simulink model "ORC_test_simu_unregSCIG"  (R2018a)
settings: Solver=FixedStepAuto  StartTime=0.0  StopTime=10  FixedStep=.1  RelTol=1e-4
values from neighbouring files (symbols this model uses):
  A_cond = 50    [Chena_ORC_test_simu_init.m]    (also in ORC_test_simu_init.m = 18.6)
  A_evap = 30    [Chena_ORC_test_simu_init.m]    (also in ORC_test_simu_init.m = 9.3)
  Cx = 620e-05    (= 0.0062)    [Chena_ORC_test_simu_init.m]    (also in ORC_test_simu_init.m = 0.000221048532072; SCIG_Admittance_Balance.m = 6.9e-05; SCIG_Energy_Balance_excitation.m = 1.35135135135; SCIG_Energy_Balance_excitation_sym.m = 5)
  eff_inverter = 0.93    [Chena_ORC_test_simu_init.m]    (also in ORC_test_simu_init.m)
  eff_pump = 0.78    [Chena_ORC_test_simu_init.m]    (also in ORC_Energy_Balance.m = 0.7; ORC_test.m = 0.7; ORC_test_brownfield.m = 0.7; ORC_test_greenfield.m = 0.7)
  eff_turbine = 0.8    [Chena_ORC_test_simu_init.m]    (also in ORC_test_simu_init.m = 0.78)
  f_rated = 60    [Chena_ORC_test_simu_init.m]    (also in ORC_test_simu_init.m; SCIG_Admittance_Balance.m; SCIG_Admittance_test.m; SCIG_Ouazenne.m)
  H_wf_init = 2.6e+05    (= 260000)    [Chena_ORC_test_simu_init.m]    (also in ORC_test_simu_init.m = 230000)
  Lr = 0.252/(2*pi*f_rated)/35    (= 1.9098593171e-05)    [Chena_ORC_test_simu_init.m]    (also in ORC_test_simu_init.m = 0.000132629119243)
  Ls = 0.423/(2*pi*f_rated)/35    (= 3.20583528228e-05)    [Chena_ORC_test_simu_init.m]    (also in ORC_test_simu_init.m = 0.000848826363157)
  m_dot_source = 33.39    [Chena_ORC_test_simu_init.m]    (also in ORC_Energy_Balance.m = 5.7714; ORC_test.m = 12; ORC_test_brownfield.m = 6; ORC_test_greenfield.m = 12)
  m_dot_wf_init = 12    [Chena_ORC_test_simu_init.m]    (also in ORC_test_simu_init.m = 3)
  m_dot_wf_max = 16    [Chena_ORC_test_simu_init.m]
  magCurveV = [98.1532063054068,98.8036071709152,99.4518999785459,100.098037520928,100.741973127402,101.383660677656,102.023054614968,102.660109959042,103.294782318460,103.927027902737,104.556803533993,105.184066658235,105.808775356268,106.430888354220,107.050365033694,107.667165441552,108.281250299330,108.892581012284,109.501119678081,110.106829095126,110.709672770539,111.309614927775,111.906620513896,112.5006 ...(+6146 chars)    [Chena_ORC_test_simu_init.m]    (also in ORC_test_simu_init.m = [21.5410077151772,22.1687511430959,22.7961934111159,23.42344)
  magCurveX = [0.663529769645709,0.663521969965503,0.663500208426959,0.663464444749194,0.663414643227627,0.663350772676200,0.663272806369214,0.663180721982808,0.663074501536138,0.662954131332260,0.662819601898778,0.662670907928276,0.662508048218555,0.662331025612717,0.662139846939116,0.661934522951205,0.661715068267290,0.661481501310239,0.661233844247137,0.660972122928937,0.660696366830103,0.660406608988283,0.6 ...(+6531 chars)    [Chena_ORC_test_simu_init.m]    (also in ORC_test_simu_init.m = [21.5410077151772,21.5637559851946,21.5850104594817,21.60498)
  p_atm = 101325    [Chena_ORC_test_simu_init.m]    (also in ORC_test_simu_init.m)
  pf_grid = 0.9    [Chena_ORC_test_simu_init.m]    (also in ORC_test_simu_init.m)
  poles = 2    [Chena_ORC_test_simu_init.m]    (also in Copy_of_SCIG_Energy_Balance_excitation.m = 4; SCIG_Admittance_Balance.m = 6; SCIG_Admittance_test.m = 6; SCIG_Ouazenne.m)
  Rr = 0.144/35    (= 0.00411428571429)    [Chena_ORC_test_simu_init.m]    (also in ORC_test_simu_init.m = 0.03)
  Rs = 0.148/35    (= 0.00422857142857)    [Chena_ORC_test_simu_init.m]    (also in ORC_test_simu_init.m = 0.018)
  Rx = 0    [Chena_ORC_test_simu_init.m]    (also in Copy_of_SCIG_Energy_Balance_excitation.m = 0.003; ORC_test_simu_init.m; SCIG_Admittance_Balance.m; SCIG_Admittance_test.m)
  Tin_sink = 277.59    [Chena_ORC_test_simu_init.m]    (also in ORC_test_simu_init.m = 278)
  Tin_source = 346.48    [Chena_ORC_test_simu_init.m]    (also in ORC_test_simu_init.m = 368)
  U_cond = 5000    [Chena_ORC_test_simu_init.m]    (also in ORC_test_simu_init.m = 1400)
  U_evap = 4500    [Chena_ORC_test_simu_init.m]    (also in ORC_test_simu_init.m = 1500)
  Vline_rated = 220    [Chena_ORC_test_simu_init.m]    (also in SCIG_Admittance_Balance.m = 6600; SCIG_Admittance_test.m = 6600; SCIG_Ouazenne.m; SCIG_Ouazenne_iterate.m)
  Xx = 1/(2*pi*f_rated*Cx)    (= 0.427835868527)    [Chena_ORC_test_simu_init.m]    (also in Copy_of_SCIG_Energy_Balance_excitation.m = 12; ORC_test_simu_init.m = 12; SCIG_Admittance_Balance.m = Xx(fvIDX); SCIG_Energy_Balance_excitation.m = 1./(Cx.*w_synch))
undefined symbols (not defined in the file or in its folder): handle_sink, handle_source, handle_wf, n_mech_init, n_mech_max, n_mech_min, sigbuilder_block
(part 3 of 4)

== matlab function ORC_test_simu_unregSCIG/ORC/Condensor/HeatExNTU_3_cond ==
  data: T_or_H_hi input; P output; m_dot_h input; p_h input; T_or_H_ci input; m_dot_c input; p_c input; fluid_h parameter uint8; fluid_c parameter; HeatExType parameter; T_or_H_ho output; T_or_H_co output; U parameter; A parameter; T_or_H parameter boolean
function [ P, T_or_H_ho, T_or_H_co ] = HeatExNTU_3_block( T_or_H_hi, m_dot_h, p_h,  ...
    T_or_H_ci, m_dot_c, p_c, fluid_h, fluid_c, HeatExType, U, A, T_or_H )

%HeatExNTU Summary 
%   This function calculates flow and outlet temperatures of a heat exchanger
%   using the Number of Transfer Units (NTU) method as described in
%   Fundementals of Heat and Mass Transfer by F. P. Incropera, D. P.
%   DeWitt, T. L. Bergman & A. S. Lavine. The method can be used when only
%   the inlet tempertures are known as opposed to inlet and outlet
%   temperatures.
%
%   This is done by calculating effectiveness which is defined as the ratio
%   of actual heat transferred to the maximum possible heat transferred for 
%   an infinite length counter-flow heat exchanger with the given inlet
%   temperatures. The effectivenes is calculated differently depending on 
%   the geometry of exchanger but is always a function of the ratio of heat
%   capacity rates as well as the number of transfer units (NTU). The NTU
%   depends on the overall heat transfer coefficient, the heat transfer
%   area, and the smaller of the two heat capacity rates. 
%   
%   In the event of a phase change the rate of change of energy required to
%   get the fluid just beyond the point of vaporizaion or condensation is
%   calculated using the CoolProp function. Then the function is called
%   again at the new temperature and the final temperatures and heat rates
%   are calucluated using a reduced heat exhange area. I currently assume
%   the effected heat transfer area is a half of the original input. This 
%   function cannot accurately handle both fluids changing phase because it
%   does not check which fluid would change first.
% 
% Note: The effectiveness is separte from efficiency. The calculations
%   assumes an efficiency of 1 where all heat is transferred from the hot
%   fluid to the cool fluid or remains within the the fluid. This also
%   assumes no fluid is undergoing a change in state, which may not be
%   sufficient for my final model.
%
% This function makes use of CoolProp, a shared DLL. 
% More information about the Matlab wrapper can be found at
%   http://www.coolprop.org/coolprop/wrappers/MATLAB/index.html
% A list of parameters can be found at 
%   http://www.coolprop.org/coolprop/HighLevelAPI.html#parameter-table
% A list of fluids can be found at 
%   http://www.coolprop.org/fluid_properties/PurePseudoPure.html#list-of-fluids
%
% Inputs:
%   T_or_H_hi   Hot fluid inlet temperature in Kelvin or enthalpy in J/kg
%   m_dot_h     Hot fluid mass flow rate in kg/s
%   p_h         Hot fluid pressure in pa
%   fluid_h     Name of Hot fluid (string)
%   T_or_H_ci   Cool fluid inlet temperature in Kelvin or enthalpy in J/kg
%   m_dot_c     Cool fluid mass flow rate in kg/s
%   p_c         Cool fluid pressure in pa
%   fluid_c     Name of Cool fluid (string)
%   HeatExType  String describing the heat exchanger geometry. Currently
%               this variable only accepts 'counter' and 'parallel', but
%               can be expanded to other exchanger/flow types
%               'counter' for counter flow
%               'parallel' for parallel
%   U           Overall heat transfer coefficient in W/(K m2)
%   A           Heat transfer area in m2
%   T_or_H      String stating whether arguements 1&5 are temperature (T) 
%               or enthaply (H). Also applies to output
%
% Output:
%   P           Rate of heat exchenged (power) in W
%   T_or_H_ho   Hot fluid outlet temperature (K) or enthalpy J/kg
%   T_or_H_co   Cool fluid outlet temperature (K) or enthalpy J/kg

% initailize certain parameters used to call coolprop library
buffer_size = 255;
ierr = 0;
b = (1:1:buffer_size);
herr= char(b);
coder.extrinsic('calllib') 
coder.extrinsic('libpointer') 

% All the input signals should be the same size, so it shouldn't matter
% which one is used to obtain signal length
var_length = length(T_or_H_hi);
% T_or_H_hi

% fluid_h = 'water';
% fluid_c = 'R245fa';
% % initialize handles for hot and cool fluids
% [fluid_h, ~] = calllib('coolprop','AbstractState_factory',backend,fluid_h,ierr,herr,buffer_size);
% [fluid_c, ~] = calllib('coolprop','AbstractState_factory',backend,fluid_c,ierr,herr,buffer_size);

% determine input parameter pair indecies for coolprop calls
[pq_ind,~] = calllib('coolprop','get_input_pair_index','PQ_INPUTS'); %pressure and Mass vapor quality
[pt_ind,~] = calllib('coolprop','get_input_pair_index','PT_INPUTS'); %pressure and temperature
[hp_ind,~] = calllib('coolprop','get_input_pair_index','HmassP_INPUTS'); %Mass specific enthalpy and pressure

% determine output parameter indecies for coolprop calls
[t_ind, ~] = calllib('coolprop','get_param_index','T'); %temperature
[h_ind, ~] = calllib('coolprop','get_param_index','Hmass'); %Mass specific enthalpy
[c_ind, ~] = calllib('coolprop','get_param_index','Cpmass'); %Mass specific constant pressure specific heat

% find pointer location of pressure and temperature input values
p_h_Ptr = libpointer('doublePtr',p_h);
p_c_Ptr = libpointer('doublePtr',p_c);
% Thi_Ptr
% Tci_Ptr
% Hhi_Ptr
% Hci_Ptr

% initialize output to zeros of appropriate length. It is necessary to
% assign output variables before recursively calling this function.
T_or_H_ho = zeros(var_length,1);
T_or_H_co = zeros(var_length,1);
% P = zeros(size(T_or_H_hi));

% disp(T_or_H )
% Ensure temperature/enthalpy input variables are delt with appropriately
% if upper(T_or_H) == 'T' %|| 'TEMPERATURE'
if T_or_H %== 'T' %|| 'TEMPERATURE'
% Assume given temperature values are not at vaporization/condensation
% disp('Assuming Temperature input')
% Initialize T and H values 
    Thi = T_or_H_hi;
    Tci = T_or_H_ci;
    Thi_Ptr = libpointer('doublePtr',Thi);
    Tci_Ptr = libpointer('doublePtr',Tci);
    Hhi = zeros(var_length,1); % initialized to 0 temporarily
    Hci = zeros(var_length,1); % initialized to 0 temporarily
    Hhi_Ptr = libpointer('doublePtr',Hhi);
    Hci_Ptr = libpointer('doublePtr',Hci);
    
% Update values located at Hhi and Hci pointer locations
    calllib('coolprop','AbstractState_update_and_1_out', fluid_h, pt_ind, p_h_Ptr, Thi_Ptr, var_length, h_ind, Hhi_Ptr, ierr,herr,buffer_size);
    calllib('coolprop','AbstractState_update_and_1_out', fluid_c, pt_ind, p_c_Ptr, Tci_Ptr, var_length, h_ind, Hci_Ptr, ierr,herr,buffer_size);
% Set Hhi & Hci to values stored at pointer location
    Hhi = get(Hhi_Ptr,'Value');
    Hci = get(Hci_Ptr,'Value');

% elseif upper(T_or_H) == 'H' %|| 'ENTHALPY'
else%if T_or_H == 'H' %|| 'ENTHALPY'
% Enthalpy values can be in vaporization/condensation region    
% disp('Assuming Enthalpy input')
% Initialize H and T values
    Hhi = T_or_H_hi;
    Hci = T_or_H_ci;
    Hhi_Ptr = libpointer('doublePtr',Hhi);
    Hci_Ptr = libpointer('doublePtr',Hci);
    Thi = zeros(var_length,1); %initialized to 0 temporarily
    Tci = zeros(var_length,1); %initialized to 0 temporarily
    Thi_Ptr = libpointer('doublePtr',Thi);
    Tci_Ptr = libpointer('doublePtr',Tci);

% Update values located at Thi and Tci pointer locations
    calllib('coolprop','AbstractState_update_and_1_out', fluid_h, hp_ind, Hhi_Ptr, p_h_Ptr, var_length, t_ind, Thi_Ptr, ierr,herr,buffer_size);
    calllib('coolprop','AbstractState_update_and_1_out', fluid_c, hp_ind, Hci_Ptr, p_c_Ptr, var_length, t_ind, Tci_Ptr, ierr,herr,buffer_size);
% Set Thi & Tci to values stored at pointer location
    Thi = get(Thi_Ptr,'Value');
    Tci = get(Tci_Ptr,'Value');
    
% else
%     error('Please specify whether input uses variables of Temperature or Enthalpy.')
end
    

% Determine vaporization temperature for fluids at respective pressures.
% Initialize pointer locations for fluid quality and relevant temperatures
Q_Ptr = libpointer('doublePtr', zeros(var_length,1)); % Q is specifically set to 0
Tvh = zeros(var_length,1); % initialized to 0 temporarily
Tvc = zeros(var_length,1); % initialized to 0 temporarily
Tvh_Ptr = libpointer('doublePtr', Tvh);
Tvc_Ptr = libpointer('doublePtr', Tvc);

% Update values located at the Tvc & Tvh pointer locations for vaporization
% conditions
calllib('coolprop','AbstractState_update_and_1_out', fluid_h, pq_ind, p_h_Ptr, Q_Ptr, var_length, t_ind, Tvh_Ptr, ierr,herr,buffer_size);
calllib('coolprop','AbstractState_update_and_1_out', fluid_c, pq_ind, p_c_Ptr, Q_Ptr, var_length, t_ind, Tvc_Ptr, ierr,herr,buffer_size);

% Set Tvh & Tvc to values stored at pointer location
Tvh = get(Tvh_Ptr,'Value');
Tvc = get(Tvc_Ptr,'Value');

% Determine vaporization enthalpies for fluids at respective pressures
% Min enthalpies of vaporization region for hot and cool fluids (Q = 0)
Hvh_min = zeros(var_length,1); % initialized to 0 temporarily
Hvc_min = zeros(var_length,1); % initialized to 0 temporarily
Hvh_min_Ptr = libpointer('doublePtr',Hvh_min);
Hvc_min_Ptr = libpointer('doublePtr',Hvc_min);
    
% Update values located at Hvh_max and Hvc_max pointer locations
calllib('coolprop','AbstractState_update_and_1_out', fluid_h, pq_ind, p_h_Ptr, Q_Ptr, var_length, h_ind, Hvh_min_Ptr, ierr,herr,buffer_size);
calllib('coolprop','AbstractState_update_and_1_out', fluid_c, pq_ind, p_c_Ptr, Q_Ptr, var_length, h_ind, Hvc_min_Ptr, ierr,herr,buffer_size);
% Set Hvh_max & Hvc_max to values stored at pointer location
Hvh_min = get(Hvh_min_Ptr,'Value');
Hvc_min = get(Hvc_min_Ptr,'Value');

% Max enthalpies of vaporization region for hot and cool fluid (Q = 1)
Q_Ptr = libpointer('doublePtr', ones(var_length,1)); % Q is specifically set to 1
Hvh_max = zeros(var_length,1); % initialized to 0 temporarily
Hvc_max = zeros(var_length,1); % initialized to 0 temporarily
Hvh_max_Ptr = libpointer('doublePtr',Hvh_max);
Hvc_max_Ptr = libpointer('doublePtr',Hvc_max);
    
% Update values located at Hvh_max and Hvc_max pointer locations
calllib('coolprop','AbstractState_update_and_1_out', fluid_h, pq_ind, p_h_Ptr, Q_Ptr, var_length, h_ind, Hvh_max_Ptr, ierr,herr,buffer_size);
calllib('coolprop','AbstractState_update_and_1_out', fluid_c, pq_ind, p_c_Ptr, Q_Ptr, var_length, h_ind, Hvc_max_Ptr, ierr,herr,buffer_size);
% Set Hvh_max & Hvc_max to values stored at pointer location
Hvh_max = get(Hvh_max_Ptr,'Value');
Hvc_max = get(Hvc_max_Ptr,'Value');


% Determine the specific heats of the incoming fluids using coolprop
% Initialize pointer locations for relevant variables
Ch = zeros(var_length,1); % initialized to 0 temporarily
Cc = zeros(var_length,1); % initialized to 0 temporarily
Ch_Ptr = libpointer('doublePtr', Ch); 
Cc_Ptr = libpointer('doublePtr', Cc); 

% Update values located at the Ch & Cc pointer locations for input
% conditions
calllib('coolprop','AbstractState_update_and_1_out', fluid_h, hp_ind, Hhi_Ptr, p_h_Ptr, var_length, c_ind, Ch_Ptr, ierr,herr,buffer_size);
calllib('coolprop','AbstractState_update_and_1_out', fluid_c, hp_ind, Hci_Ptr, p_c_Ptr, var_length, c_ind, Cc_Ptr, ierr,herr,buffer_size);

% Set Ch & Cc to values stored at pointer location
Ch = get(Ch_Ptr,'Value');   % J/(kg K)
Cc = get(Cc_Ptr,'Value');   % J/(kg K)

% If the fluid is withing the vaporization range then the coolprop library 
% will return an inaccurate values. If that happens then the specific heat 
% will be set to inf so its temperature will not change even though heat is
% exchanged.
Ch(Hhi <= Hvh_max & Hhi > Hvh_min) = inf;    % J/(kg K)
Cc(Hci < Hvc_max & Hci >= Hvc_min) = inf;    % J/(kg K)

% Calculate the heat capacity rates of the hot and cool fluids
Ch_rate = Ch .* m_dot_h;     % W/K
Cc_rate = Cc .* m_dot_c;     % W/K

% Determine the maximum and minimum of the two heat capacity rates
Cmax = Ch_rate; % W/K
Cmax(Ch_rate < Cc_rate) = Cc_rate(Ch_rate < Cc_rate);   % W/K
Cmin = Ch_rate; % W/K
Cmin(Ch_rate > Cc_rate) = Cc_rate(Ch_rate > Cc_rate);   % W/K

% Calcluate the heat capacity rate ratio 
Cr = Cmin./Cmax;

% unitA is the size of heat exchanger area(m2) each iteration of the script
% uses for calculating NTU
% unitA = 1;
unitA = A .* ones(var_length,1);

% Calculate the number of transfer units of the heat exchanger
if any(A < unitA)
    unitA = A .* ones(var_length,1);
%     NTU = U * A / Cmin
end

NTU = U * unitA ./ Cmin;


HeatExType = 'counter';
% Calculate effectiveness based on type of heat exchanger
switch HeatExType
    case 'counter'  % If the heat exchanger is counter-flow
        effectiveness = (1 - exp(-NTU.*(1 - Cr))) ./ ...
                        (1 - Cr.*exp(-NTU.*(1 - Cr)));
    case 'parallel' % If the heat exchanger is parallel-flow
        effectiveness = (1 - exp(-NTU.*(1 + Cr))) ./ ...
                        (1 + Cr);
    otherwise       % If not exchanger specified
%         warning('No heat exchanger type specified, therefore no heat is exchanged.')
        effectiveness = 0;
end        

% % However if the Cr is 0 (Cmax is inf) then effectiveness is calcluated
% % regardless of the heat exchanger flow.
% if Cr == 0
%     effectiveness = 1 - exp(-NTU);
% end
% effectiveness;


% Maximum energy transfer rate is equal for an infinite length heat
% exchanger is equal to Cmin multiplied with the difference in inlet
% temperatures. The actual energy transfer rate is the maximum rate
% multiplied by the effectiveness (Assuming no heat loss).
P = effectiveness.*Cmin.*(Thi - Tci);

% The change in temperature is calculated for both sides by dividing the
% energy tranfer rate by the heat capacity rates for both sides. This
% assumes the energy transfer rate is the same for both sides.
deltaTh = P./Ch_rate;
deltaTc = P./Cc_rate;

% The outlet temperatures are caluctaed by subtracting the change in
% temperature from the hot fluid inlet temperature and adding the change in
% temperature from the cool fluid inlet temperature.
Tho = Thi - deltaTh;
Tco = Tci + deltaTc;

% Determine Hho and Hco values based off of Tho and Tco values
% Initialize Hho and Hco values and pointers and Tho & Tco pointers
Tho_Ptr = libpointer('doublePtr',Tho);
Tco_Ptr = libpointer('doublePtr',Tco);
Hho = zeros(var_length,1); % initialized to 0 temporarily
Hco = zeros(var_length,1); % initialized to 0 temporarily
Hho_Ptr = libpointer('doublePtr',Hho);
Hco_Ptr = libpointer('doublePtr',Hco);
    
% Update values located at Hho and Hco pointer locations
calllib('coolprop','AbstractState_update_and_1_out', fluid_h, pt_ind, p_h_Ptr, Tho_Ptr, var_length, h_ind, Hho_Ptr, ierr,herr,buffer_size);
calllib('coolprop','AbstractState_update_and_1_out', fluid_c, pt_ind, p_c_Ptr, Tco_Ptr, var_length, h_ind, Hco_Ptr, ierr,herr,buffer_size);
% Set Hho & Hco to values stored at pointer location
Hho = get(Hho_Ptr,'Value');
Hco = get(Hco_Ptr,'Value');

% The coolprop will fail to update if Tho = vaporization temperature. In
% that case, those values will remain zero because it was initialized to 
% zero. For those values Ho = Hi - P/m_dot
Hho(~Hho) =  Hhi(~Hho) - P(~Hho)./m_dot_h(~Hho);

% The coolprop will fail to update if Tco = vaporization temperature. In
% that case, those values will remain zero because it was initialized to 
% zero. For those values Ho = Hi + P/m_dot
Hco(~Hco) =  Hci(~Hco) + P(~Hco)./m_dot_c(~Hco);


% check if hot fluid begins to condense 
if any(Hho <= Hvh_max & Hhi > Hvh_max)
% if Tho <= Tvh && Thi >= Tvh
%     disp('~~~~~~~~~~~~~~~~~~~Condensation start~~~~~~~~~~~~~~~~~~~~~')

%     Get the indecies where condensation starts
    cond_start_ind = (Hho <= Hvh_max & Hhi > Hvh_max);
    
%     Set the H output of the appropriate values to maximum value in the
%     vaporization region (Q = 1)
    Hho(cond_start_ind) = Hvh_max(cond_start_ind);
    Tho(cond_start_ind) = Tvh(cond_start_ind);
    
%     Calculate power needed to bring hot fluid initial state to
%     precondense for only relevant values
    P_init_to_precondense = (Hhi(cond_start_ind) - Hho(cond_start_ind)).*m_dot_h(cond_start_ind);

%     Calculate change in temperature for relavent cool fluid values
    deltaTc = P_init_to_precondense./Cc_rate(cond_start_ind);
%     Update relavent cool fluid output temperatures and get new pointer
    Tco(cond_start_ind) = Tci(cond_start_ind) + deltaTc;
    Tco_Ptr = libpointer('doublePtr',Tco);
    
%     Update H values for new cool output temperatures
    calllib('coolprop','AbstractState_update_and_1_out', fluid_c, pt_ind, p_c_Ptr, Tco_Ptr, var_length, h_ind, Hco_Ptr, ierr,herr,buffer_size);
    Hco = get(Hco_Ptr,'Value');

%     Calculate ratio of power to precondense state relative to initally
%     calculated power in order to correct the area of relavent values
    PowerFrac_Condense_over_NoCondense = P_init_to_precondense./P(cond_start_ind);
    unitA(cond_start_ind) = unitA(cond_start_ind)*PowerFrac_Condense_over_NoCondense;
%     Update relevant power values
    P(cond_start_ind) = P_init_to_precondense;
    
% check if hot fluid finishes condensing    
elseif any(Hho <= Hvh_min & Hhi > Hvh_min)
% elseif Tho <= Tvh && Thi >= Tvh
%     disp('~~~~~~~~~~~~~~~~~~~~~~Condensation end~~~~~~~~~~~~~~~~~~~~~~~~~')

%     Get the indecies where condensation starts
    cond_end_ind = (Hho <= Hvh_min & Hhi > Hvh_min);
    
%     Set the H output of the appropriate values to minimum value in the
%     vaporization region (Q = 0)
    Hho(cond_end_ind) = Hvh_min(cond_end_ind);
    Tho(cond_end_ind) = Tvh(cond_end_ind) - 1e-4;
    
%     Calculate power needed to bring hot fluid initial state to
%     postcondense for only relevant values
    P_init_to_postcondense = (Hhi(cond_end_ind) - Hho(cond_end_ind)).*m_dot_h(cond_end_ind);

%     Calculate change in temperature for relavent cool fluid values
    deltaTc = P_init_to_postcondense./Cc_rate(cond_end_ind);
%     Update relavent cool fluid output temperatures and get new pointer
    Tco(cond_end_ind) = Tci(cond_end_ind) + deltaTc;
    Tco_Ptr = libpointer('doublePtr',Tco);

%     Update H values for new cool output temperatures
    calllib('coolprop','AbstractState_update_and_1_out', fluid_c, pt_ind, p_c_Ptr, Tco_Ptr, var_length, h_ind, Hco_Ptr, ierr,herr,buffer_size);
    Hco = get(Hco_Ptr,'Value');

%     Calculate ratio of power to postcondense state relative to initally
%     calculated power in order to correct the area of relavent values
    PowerFrac_Condense_over_NoCondense = P_init_to_postcondense./P(cond_end_ind);
    unitA(cond_end_ind) = unitA(cond_end_ind)*PowerFrac_Condense_over_NoCondense;
%     Update relevant power values
    P(cond_end_ind) = P_init_to_postcondense;
 

% else check if cool fluid begins to vaporize
elseif any(Hco >= Hvc_min & Hci < Hvc_min)
% elseif Tco >= Tvc && Tci <= Tvc
%    disp('~~~~~~~~~~~~~~~~~~~Vaporization start~~~~~~~~~~~~~~~~~~~~~~~~')

%     Get the indecies where vaporization starts
    vap_start_ind = (Hco >= Hvc_min & Hci < Hvc_min);

%     Set the H output of the appropriate values to minimum value in the
%     vaporization region (Q = 0)
    Hco(vap_start_ind) = Hvc_min(vap_start_ind);
    Tco(vap_start_ind) = Tvc(vap_start_ind);

%     Calculate power needed to bring cool fluid initial state to
%     prevaporization for only relevant values
    P_init_to_prevap = (Hco(vap_start_ind) - Hci(vap_start_ind)).*m_dot_c(vap_start_ind);

%     Calculate change in temperature for relavent hot fluid values
    deltaTh = P_init_to_prevap./Ch_rate(vap_start_ind);
%     Update relavent hot fluid output temperatures and get new pointer
    Tho(vap_start_ind) = Thi(vap_start_ind) - deltaTh;
    Tho_Ptr = libpointer('doublePtr',Tho);

%     Update H values for new hot output temperatures
    calllib('coolprop','AbstractState_update_and_1_out', fluid_h, pt_ind, p_h_Ptr, Tho_Ptr, var_length, h_ind, Hho_Ptr, ierr,herr,buffer_size);
    Hho = get(Hho_Ptr,'Value');

%     Calculate ratio of power to prevaporize state relative to initally
%     calculated power in order to correct the area of relavent values
    PowerFrac_Vaporize_over_NoVaporize = P_init_to_prevap./P(vap_start_ind);
    unitA(vap_start_ind) = unitA(vap_start_ind).*PowerFrac_Vaporize_over_NoVaporize;
%     Update relevant power values
    P(vap_start_ind) = P_init_to_prevap;

    
% check if cool fluid finishes vaporizing
elseif any(Hco >= Hvc_max & Hci < Hvc_max)
% elseif Tho <= Tvh && Thi >= Tvh
%     disp('~~~~~~~~~~~~~~~~Vaporization end~~~~~~~~~~~~~~~~~~~~')

%     Get the indecies where vaporization ends
    vap_end_ind = (Hco >= Hvc_max & Hci < Hvc_max);

%     Set the H output of the appropriate values to maximum value in the
%     vaporization region (Q = 1)
    Hco(vap_end_ind) = Hvc_max(vap_end_ind);
    Tco(vap_end_ind) = Tvc(vap_end_ind) + 1e-4;

%     Calculate power needed to bring cool fluid initial state to
%     postvaporization for only relevant values
    P_init_to_postvap = (Hco(vap_end_ind) - Hci(vap_end_ind)).*m_dot_c(vap_end_ind);

%     Calculate change in temperature for relavent hot fluid values
    deltaTh = P_init_to_postvap./Ch_rate(vap_end_ind);
%     Update relavent hot fluid output temperatures and get new pointer
    Tho(vap_end_ind) = Thi(vap_end_ind) - deltaTh;
    Tho_Ptr = libpointer('doublePtr',Tho);

%     Update H values for new hot output temperatures
    calllib('coolprop','AbstractState_update_and_1_out', fluid_h, pt_ind, p_h_Ptr, Tho_Ptr, var_length, h_ind, Hho_Ptr, ierr,herr,buffer_size);
    Hho = get(Hho_Ptr,'Value');

%     Calculate ratio of power to prevaporize state relative to initally
%     calculated power in order to correct the area of relavent values
    PowerFrac_Vaporize_over_NoVaporize = P_init_to_postvap./P(vap_end_ind);
    unitA(vap_end_ind) = unitA(vap_end_ind).*PowerFrac_Vaporize_over_NoVaporize;
%     Update relevant power values
    P(vap_end_ind) = P_init_to_postvap;

else
%     disp('~~~~~~~~~~~~~~~~Maintain State~~~~~~~~~~~~~~~~~~~~')
end
%     Hhi
%     Hho
%     Thi
%     Tho
%     Hci
%     Hco
%     Tci
%     Tco
%     P

% double check if hot fluid would condense and cool fluid would vaporize
if any((Tho < Tvh & Thi > Tvh) & (Tco > Tvc & Tci < Tvc))
    error('This function cannot accurately handle both fluids changing phase.')
end

if A > unitA

%     P_next = zeros(size(T_or_H_hi));
%     disp(P)
    [ P_next, Hho, Hco ] = HeatExNTU_3_low( Hho, m_dot_h, p_h, ...
        Hco, m_dot_c, p_c, fluid_h, fluid_c, HeatExType, U, A - unitA, 'H' );
%     A
%     unitA
% %     A - unitA;
%     P_next
    P = P + P_next;
%     disp(['Power After: ' num2str(P) ' W'])

    Hho_Ptr = libpointer('doublePtr',Hho);
    Hco_Ptr = libpointer('doublePtr',Hco);
% Update values located at Tho and Tco pointer locations
    calllib('coolprop','AbstractState_update_and_1_out', fluid_h, hp_ind, Hho_Ptr, p_h_Ptr, var_length, t_ind, Tho_Ptr, ierr,herr,buffer_size);
    calllib('coolprop','AbstractState_update_and_1_out', fluid_c, hp_ind, Hco_Ptr, p_c_Ptr, var_length, t_ind, Tco_Ptr, ierr,herr,buffer_size);
% Set Thi & Tci to values stored at pointer location
    Tho = get(Tho_Ptr,'Value');
    Tco = get(Tco_Ptr,'Value');

else
%     P
end


% % Free the hot and cool fluid handles
% calllib('coolprop','AbstractState_free', fluid_h, ierr,herr,buffer_size);
% calllib('coolprop','AbstractState_free', fluid_c, ierr,herr,buffer_size);

% if upper(T_or_H) == 'T' %|| 'TEMPERATURE'
if T_or_H% == 'T' %|| 'TEMPERATURE'
    T_or_H_ho = Tho;
    T_or_H_co = Tco;
% elseif upper(T_or_H) == 'H' %|| 'ENTHALPY'
else%if T_or_H == 'H' %|| 'ENTHALPY'
    T_or_H_ho = Hho;
    T_or_H_co = Hco;
end
end

== matlab function ORC_test_simu_unregSCIG/ORC/Pump/IsentropicPower_pump ==
  data: T_or_H_i input; P_hy output; p_i input; p_o input; m_dot input; T_or_H_o output; T_or_H parameter; isen_eff parameter; fluid parameter
function [ P_hy, T_or_H_o ] = IsentropicPower_block( T_or_H_i, p_i, p_o, m_dot, T_or_H,  isen_eff, fluid)
% function [ P_hy ] = IsentropicPower( T_i, T_o, p_i, p_o, m_dot, fluid, isen_eff )
%EXPANDER Summary of this function
%   This process calculates the mechanical power provided or required by a 
%   generic expander device/system. Turbines and other expanders provide
%   mechanical power while pumps and compressors consume it. This is done
%   by calculating the change in enthalpy of fluid and multipying by the 
%   mass flow rate while entropy remains constant.  Non ideal processes are
%   taken into account through the isentropic efficiency.
% 
% Inputs:
%   T_or_H_i    Input temperature in Kelvin or enthalpy in J/kg
%   p_i         Input pressure of the fluid in Pa
%   p_o         Output temperature of the fluid in Pa
%   m_dot       Mass flow rate of the fluid in kg/s 
%   fluid       Initialzed coolprop fluid handle
%   isen_eff    Isentropic efficiency of the device. Expected range: 0-1
%               This input is optional. If it is not provided then it will 
%               be set to 1, which is the efficiency of an ideal isentropic
%               device where entropy is constant.
%               This value is treated differently depending on if there is
%               an increase or decrease in fluid enthalpy. If the enthalpy
%               decreases (energy is extracted from the system) then the
%               efficiency if multiplied by the change in energy because
%               less energy is extracted than the ideal case. If the
%               enthalpy increases (energy in added to the system) then the
%               efficiency is divided by the change in energy because more
%               energy is required than the ideal case.
%   T_or_H      Logical indicating whether the relavent input and output
%               variables are temperature (1) or enthalpy (0)
% 
% Outputs:
%   P_hy        Hydraulic power exctracted or consumed in W. Positive
%               values indicate the system is providing hydraulic power as
%               a turbine or expander. Negative values indicate the system 
%               is consuming hydraulic power as a compressor or pump.
%   T_or_H_o    Output temperature in Kelvin or enthalpy in J/kg

% This function makes use of the CoolProp wrapper for fluid properties. 
% The high level Matlab wrapper cannot handle vector inputs. There ways to
% make low level calls interfacing with the DLL so many values can be
% determined more quickly, but that is not implented here.
% More information about the Matlab wrapper can be found at
%   http://www.coolprop.org/coolprop/wrappers/MATLAB/index.html
% A list of parameters can be found at 
%   http://www.coolprop.org/coolprop/HighLevelAPI.html#parameter-table
% A list of fluids can be found at 
%   http://www.coolprop.org/fluid_properties/PurePseudoPure.html#list-of-fluids

% initailize certain parameters used to call coolprop library
buffer_size = 255;
ierr = 0;
b = (1:1:buffer_size);
herr= char(b);
coder.extrinsic('calllib') 
coder.extrinsic('libpointer') 

% All the input signals should be the same size, so it shouldn't matter
% which one is used to obtain signal length
var_length = length(T_or_H_i);

% determine input parameter pair indecies for coolprop calls
% [pq_ind,~] = calllib('coolprop','get_input_pair_index','PQ_INPUTS'); %pressure and Mass vapor quality
[pt_ind,~] = calllib('coolprop','get_input_pair_index','PT_INPUTS'); %pressure and temperature
[hp_ind,~] = calllib('coolprop','get_input_pair_index','HmassP_INPUTS'); %Mass specific enthalpy and pressure
[ps_ind,~] = calllib('coolprop','get_input_pair_index','PSmass_INPUTS'); %pressure and Mass specific entropy

% determine output parameter indecies for coolprop calls
[t_ind, ~] = calllib('coolprop','get_param_index','T'); %temperature
[s_ind, ~] = calllib('coolprop','get_param_index','S'); %Mass specific entropy
[h_ind, ~] = calllib('coolprop','get_param_index','Hmass'); %Mass specific enthalpy
% [c_ind, ~] = calllib('coolprop','get_param_index','Cpmass'); %Mass specific constant pressure specific heat

% find pointer location of pressure input and output values
p_i_Ptr = libpointer('doublePtr',p_i);
p_o_Ptr = libpointer('doublePtr',p_o);

% Ensure temperature/enthalpy input variables are delt with appropriately
if T_or_H 
% Assume given temperature values are not at vaporization/condensation.
% Initialize T and H inputs
    T_i = T_or_H_i;
    T_i_Ptr = libpointer('doublePtr',T_i);
    H_i = zeros(var_length,1); % initialized to 0 temporarily
    H_i_Ptr = libpointer('doublePtr',H_i);
% Update values located at Hhi and Hci pointer locations
    calllib('coolprop','AbstractState_update_and_1_out', fluid, pt_ind, p_i_Ptr, T_i_Ptr, var_length, h_ind, H_i_Ptr, ierr,herr,buffer_size);
% Set Hhi & Hci to values stored at pointer location
    H_i = get(H_i_Ptr,'Value');
    
else
% Enthalpy values can be in vaporization/condensation region  
% Initialize H values
    H_i = T_or_H_i;
    H_i_Ptr = libpointer('doublePtr',H_i);

end

% Input entropy in J/kg/K
% Initialize pointer locations for relevant variables
S_i_Ptr = libpointer('doublePtr', zeros(var_length,1)); 
% Update values at S_i pointer location
calllib('coolprop','AbstractState_update_and_1_out', fluid, hp_ind, H_i_Ptr, p_i_Ptr, var_length, s_ind, S_i_Ptr, ierr,herr,buffer_size);
% Set S_i to values stored at pointer location
% S_i = get(S_i_Ptr,'Value');

% Ideal Output entropy is equal to input entropy 
% Ideal Output enthalpy in J/kg and temperature
H_o_ideal = zeros(var_length,1);
H_o_ideal_Ptr = libpointer('doublePtr',H_o_ideal);
% Update values located at Hhi and Hci pointer locations
calllib('coolprop','AbstractState_update_and_1_out', fluid, ps_ind, p_o_Ptr, S_i_Ptr, var_length, h_ind, H_o_ideal_Ptr, ierr,herr,buffer_size);
% Set H_o_ideal to values stored at pointer location
H_o_ideal = get(H_o_ideal_Ptr,'Value');

% Calculate Ideal power consumed/provided
P_ideal = m_dot.*(H_i - H_o_ideal);

% Initialize hydrolic power variable
P_hy = zeros(var_length,1);
%   If positive then the system is providing power as a turbine
%   or expander.
%   This means the actual power provided is less than the ideal power
P_hy(P_ideal > 0) = isen_eff.*P_ideal(P_ideal > 0);

%   If negative then the system is consuming power as a
%   compressor or pump.
%   This means the actual power consumed is greater than the ideal power.
P_hy(P_ideal < 0) = P_ideal(P_ideal < 0)./isen_eff;

% Set output enthalpy
H_o = H_i - P_hy./m_dot;
H_o_Ptr = libpointer('doublePtr',H_o);

% Ensure temperature/enthalpy input variables are delt with appropriately
if T_or_H 
% Assume given temperature values are not at vaporization/condensation
    T_or_H_o = zeros(var_length,1);
    T_or_H_o_Ptr = libpointer('doublePtr',T_or_H_o);
    calllib('coolprop','AbstractState_update_and_1_out', fluid, hp_ind, H_o_Ptr, p_o_Ptr, var_length, t_ind, T_or_H_o_Ptr, ierr,herr,buffer_size);
    T_or_H_o = get(T_or_H_o_Ptr,'Value');
    
else
% Enthalpy values can be in vaporization/condensation region    
    T_or_H_o = H_o;
end
end

== matlab function ORC_test_simu_unregSCIG/ORC/hp2t ==
  data: temperature output; enthalpy input; pressure input; fluid_handle parameter
function temperature  = hp2t(enthalpy,pressure, fluid_handle)
%HP2T Summary of this function goes here
%   This function takes caluculates the temperature of a fluid based off of
%   its enthalpy and pressure using the Cool Prob library. The fluid handle
%   must already be generated and input in order to calculate the output
%   values.

buffer_size = 255;
ierr = 0;
b = (1:1:buffer_size);
herr= char(b);
coder.extrinsic('calllib') 
coder.extrinsic('libpointer') 

[hp_ind,~] = calllib('coolprop','get_input_pair_index','HmassP_INPUTS'); %Mass specific enthalpy and pressure
[t_ind, ~] = calllib('coolprop','get_param_index','T'); %temperature

var_len = length(pressure);
pressurePtr = libpointer('doublePtr',pressure);
enthaplyPtr = libpointer('doublePtr',enthalpy);
temperature = zeros(var_len,1);
temperaturePtr = libpointer('doublePtr',temperature);

calllib('coolprop','AbstractState_update_and_1_out', fluid_handle, hp_ind, enthaplyPtr, pressurePtr, var_len, t_ind, temperaturePtr, ierr,herr,buffer_size);

temperature = get(temperaturePtr,'Value');

end

== matlab function ORC_test_simu_unregSCIG/ORC/hp2t1 ==
  data: temperature output; enthalpy input; pressure input; fluid_handle parameter
function temperature  = hp2t(enthalpy,pressure, fluid_handle)
%HP2T Summary of this function goes here
%   This function takes caluculates the temperature of a fluid based off of
%   its enthalpy and pressure using the Cool Prob library. The fluid handle
%   must already be generated and input in order to calculate the output
%   values.

buffer_size = 255;
ierr = 0;
b = (1:1:buffer_size);
herr= char(b);
coder.extrinsic('calllib') 
coder.extrinsic('libpointer') 

[hp_ind,~] = calllib('coolprop','get_input_pair_index','HmassP_INPUTS'); %Mass specific enthalpy and pressure
[t_ind, ~] = calllib('coolprop','get_param_index','T'); %temperature

var_len = length(pressure);
pressurePtr = libpointer('doublePtr',pressure);
enthaplyPtr = libpointer('doublePtr',enthalpy);
temperature = zeros(var_len,1);
temperaturePtr = libpointer('doublePtr',temperature);

calllib('coolprop','AbstractState_update_and_1_out', fluid_handle, hp_ind, enthaplyPtr, pressurePtr, var_len, t_ind, temperaturePtr, ierr,herr,buffer_size);

temperature = get(temperaturePtr,'Value');

end

== matlab function ORC_test_simu_unregSCIG/ORC/hp2t2 ==
  data: temperature output; enthalpy input; pressure input; fluid_handle parameter
function temperature  = hp2t(enthalpy,pressure, fluid_handle)
%HP2T Summary of this function goes here
%   This function takes caluculates the temperature of a fluid based off of
%   its enthalpy and pressure using the Cool Prob library. The fluid handle
%   must already be generated and input in order to calculate the output
%   values.

buffer_size = 255;
ierr = 0;
b = (1:1:buffer_size);
herr= char(b);
coder.extrinsic('calllib') 
coder.extrinsic('libpointer') 

[hp_ind,~] = calllib('coolprop','get_input_pair_index','HmassP_INPUTS'); %Mass specific enthalpy and pressure
[t_ind, ~] = calllib('coolprop','get_param_index','T'); %temperature

var_len = length(pressure);
pressurePtr = libpointer('doublePtr',pressure);
enthaplyPtr = libpointer('doublePtr',enthalpy);
temperature = zeros(var_len,1);
temperaturePtr = libpointer('doublePtr',temperature);

calllib('coolprop','AbstractState_update_and_1_out', fluid_handle, hp_ind, enthaplyPtr, pressurePtr, var_len, t_ind, temperaturePtr, ierr,herr,buffer_size);

temperature = get(temperaturePtr,'Value');

end

== matlab function ORC_test_simu_unregSCIG/ORC/hp2t3 ==
  data: temperature output; enthalpy input; pressure input; fluid_handle parameter
function temperature  = hp2t(enthalpy,pressure, fluid_handle)
%HP2T Summary of this function goes here
%   This function takes caluculates the temperature of a fluid based off of
%   its enthalpy and pressure using the Cool Prob library. The fluid handle
%   must already be generated and input in order to calculate the output
%   values.

buffer_size = 255;
ierr = 0;
b = (1:1:buffer_size);
herr= char(b);
coder.extrinsic('calllib') 
coder.extrinsic('libpointer') 

[hp_ind,~] = calllib('coolprop','get_input_pair_index','HmassP_INPUTS'); %Mass specific enthalpy and pressure
[t_ind, ~] = calllib('coolprop','get_param_index','T'); %temperature

var_len = length(pressure);
pressurePtr = libpointer('doublePtr',pressure);
enthaplyPtr = libpointer('doublePtr',enthalpy);
temperature = zeros(var_len,1);
temperaturePtr = libpointer('doublePtr',temperature);

calllib('coolprop','AbstractState_update_and_1_out', fluid_handle, hp_ind, enthaplyPtr, pressurePtr, var_len, t_ind, temperaturePtr, ierr,herr,buffer_size);

temperature = get(temperaturePtr,'Value');

end

== matlab function ORC_test_simu_unregSCIG/ORC/hp2t4 ==
  data: temperature output; enthalpy input; pressure input; fluid_handle parameter
function temperature  = hp2t(enthalpy,pressure, fluid_handle)
%HP2T Summary of this function goes here
%   This function takes caluculates the temperature of a fluid based off of
%   its enthalpy and pressure using the Cool Prob library. The fluid handle
%   must already be generated and input in order to calculate the output
%   values.

buffer_size = 255;
ierr = 0;
b = (1:1:buffer_size);
herr= char(b);
coder.extrinsic('calllib') 
coder.extrinsic('libpointer') 

[hp_ind,~] = calllib('coolprop','get_input_pair_index','HmassP_INPUTS'); %Mass specific enthalpy and pressure
[t_ind, ~] = calllib('coolprop','get_param_index','T'); %temperature

var_len = length(pressure);
pressurePtr = libpointer('doublePtr',pressure);
enthaplyPtr = libpointer('doublePtr',enthalpy);
temperature = zeros(var_len,1);
temperaturePtr = libpointer('doublePtr',temperature);

calllib('coolprop','AbstractState_update_and_1_out', fluid_handle, hp_ind, enthaplyPtr, pressurePtr, var_len, t_ind, temperaturePtr, ierr,herr,buffer_size);

temperature = get(temperaturePtr,'Value');

end

== matlab function ORC_test_simu_unregSCIG/ORC/hp2t5 ==
  data: temperature output; enthalpy input; pressure input; fluid_handle parameter
function temperature  = hp2t(enthalpy,pressure, fluid_handle)
%HP2T Summary of this function goes here
%   This function takes caluculates the temperature of a fluid based off of
%   its enthalpy and pressure using the Cool Prob library. The fluid handle
%   must already be generated and input in order to calculate the output
%   values.

buffer_size = 255;
ierr = 0;
b = (1:1:buffer_size);
herr= char(b);
coder.extrinsic('calllib') 
coder.extrinsic('libpointer') 

[hp_ind,~] = calllib('coolprop','get_input_pair_index','HmassP_INPUTS'); %Mass specific enthalpy and pressure
[t_ind, ~] = calllib('coolprop','get_param_index','T'); %temperature

var_len = length(pressure);
pressurePtr = libpointer('doublePtr',pressure);
enthaplyPtr = libpointer('doublePtr',enthalpy);
temperature = zeros(var_len,1);
temperaturePtr = libpointer('doublePtr',temperature);

calllib('coolprop','AbstractState_update_and_1_out', fluid_handle, hp_ind, enthaplyPtr, pressurePtr, var_len, t_ind, temperaturePtr, ierr,herr,buffer_size);

temperature = get(temperaturePtr,'Value');

end

== matlab function ORC_test_simu_unregSCIG/ORC/pt2h ==
  data: fluid_handle parameter; pressure input; enthalpy output; temperature input
function enthalpy  = pt2h(fluid_handle,pressure,temperature)
%PT2H Summary of this function goes here
%   This function takes caluculates the enthalpy of a fluid based off of
%   its temperature and pressure using the Cool Prob library. The fluid 
%   handle must already be generated and input in order to calculate the 
%   output values.

buffer_size = 255;
ierr = 0;
b = (1:1:buffer_size);
herr= char(b);
coder.extrinsic('calllib') 
coder.extrinsic('libpointer') 

[pt_ind,~] = calllib('coolprop','get_input_pair_index','PT_INPUTS'); %Mass specific enthalpy and pressure
[h_ind, ~] = calllib('coolprop','get_param_index','Hmass'); %temperature

var_len = length(pressure);
pressurePtr = libpointer('doublePtr',pressure);
temperaturePtr  = libpointer('doublePtr',temperature);
enthalpy = zeros(var_len,1);
enthaplyPtr = libpointer('doublePtr',enthalpy);

calllib('coolprop','AbstractState_update_and_1_out', fluid_handle, pt_ind, pressurePtr, temperaturePtr, var_len, h_ind, enthaplyPtr, ierr,herr,buffer_size);

enthalpy = get(enthaplyPtr,'Value');

end

== matlab function ORC_test_simu_unregSCIG/ORC/pt2h2 ==
  data: fluid_handle parameter; pressure input; enthalpy output; temperature input
function enthalpy  = pt2h(fluid_handle,pressure,temperature)
%PT2H Summary of this function goes here
%   This function takes caluculates the enthalpy of a fluid based off of
%   its temperature and pressure using the Cool Prob library. The fluid 
%   handle must already be generated and input in order to calculate the 
%   output values.

buffer_size = 255;
ierr = 0;
b = (1:1:buffer_size);
herr= char(b);
coder.extrinsic('calllib') 
coder.extrinsic('libpointer') 

[pt_ind,~] = calllib('coolprop','get_input_pair_index','PT_INPUTS'); %Mass specific enthalpy and pressure
[h_ind, ~] = calllib('coolprop','get_param_index','Hmass'); %temperature

var_len = length(pressure);
pressurePtr = libpointer('doublePtr',pressure);
temperaturePtr  = libpointer('doublePtr',temperature);
enthalpy = zeros(var_len,1);
enthaplyPtr = libpointer('doublePtr',enthalpy);

calllib('coolprop','AbstractState_update_and_1_out', fluid_handle, pt_ind, pressurePtr, temperaturePtr, var_len, h_ind, enthaplyPtr, ierr,herr,buffer_size);

enthalpy = get(enthaplyPtr,'Value');

end

== matlab function ORC_test_simu_unregSCIG/Inverter ==
  data: eff input; Pin input; Pout output; Ploss output
function [ Pout, Ploss ] = Inverter_Simple(eff, Pin)
% function [ Pdc, Ploss ] = Voltage_Source_Inverter_Simple(Pload, Qload, Vdc, Vac, eff, method_flag )
                            
%INVERTER Summary of this function goes here
%   This function simulates a very simple three phase voltage source 
%   inverter for an energy balance microgrid model. For a given load, input
%   and output voltage levels, and efficiency, the scripts will calculated
%   the power comsumptions seen by the DC source as well as the power loss
%   in the inverter.

% Active Power out = Active Power in * efficiency
Pout = Pin.*eff;

% loss is the difference in power
Ploss = Pin - Pout;

end
